simulink model "GalacticSoupFunctional"  (R2025b)
settings: Solver=VariableStepAuto  StartTime=0.0  StopTime=10.0  RelTol=1e-3
settings Model: DataDictionary=GalacticSoupFunctionalInterfaces.sldd  Creator=sarah  LastModifiedBy=sarah

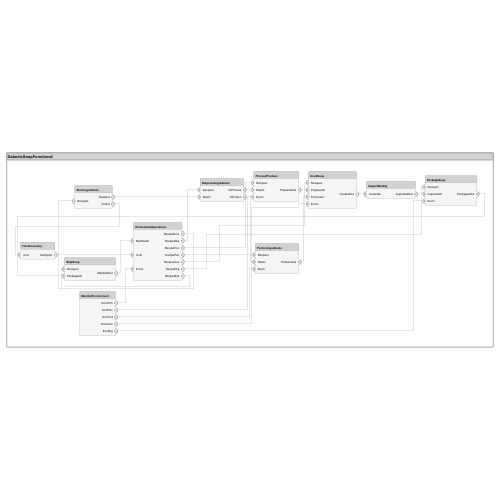
[thumbnail: Simulink's stored preview of the top-level diagram]
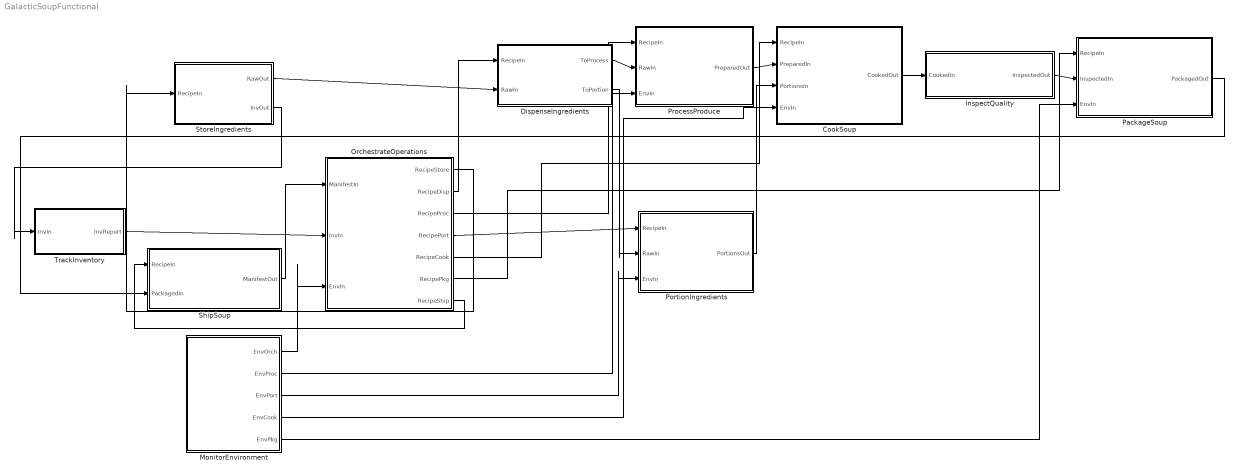
== system GalacticSoupFunctional ==
  CookSoup : Subsystem
      settings: PortSchema="{\"entries\":[{\"content\":{\"headerSize\":26,\"margin\":15,\"minimumSpacing\":25,\"sides\":[{\"content\":{\"connectorIds\":[\"In1\",\"In2\",\"In3\",\"In4\"]},\"type\":\"ConnectorPlacement.EquallySpacedRectSide\",\"uuid\":\"e444b18e-2ceb-4425-8803-e6c31b1fcd82\"},{\"content\":{\"connectorIds\":[\"Out1\"],\"side\":\"RIGHT\"},\"type\":\"ConnectorPlacement.EquallySpacedRectSide\",\"uuid\":\"f4aec6c9-b52d-4884-9c27-2bb07598a416\"},{\"content\":{\"side\":\"TOP\"},\"type\":\"ConnectorPlacement.EquallySpacedRectSide\",\"uuid\":\"1037694d-1bab-41f9-830b-c4a2d0bddcad\"}]},\"type\":\"ConnectorPlacement.EquallySpacedConnector\",\"uuid\":\"fcfa453c-694a-4044-b0a2-73b33e092223\"}],\"packageUris\":[\"http://schema.mathworks.com/mf0/Connector/R2020b\"],\"version\":\"1.0\"}"
  DispenseIngredients : Subsystem
      settings: PortSchema="{\"entries\":[{\"content\":{\"headerSize\":26,\"margin\":15,\"minimumSpacing\":25,\"sides\":[{\"content\":{\"connectorIds\":[\"In1\",\"In2\"]},\"type\":\"ConnectorPlacement.EquallySpacedRectSide\",\"uuid\":\"e444b18e-2ceb-4425-8803-e6c31b1fcd82\"},{\"content\":{\"connectorIds\":[\"Out1\",\"Out2\"],\"side\":\"RIGHT\"},\"type\":\"ConnectorPlacement.EquallySpacedRectSide\",\"uuid\":\"f4aec6c9-b52d-4884-9c27-2bb07598a416\"},{\"content\":{\"side\":\"TOP\"},\"type\":\"ConnectorPlacement.EquallySpacedRectSide\",\"uuid\":\"1037694d-1bab-41f9-830b-c4a2d0bddcad\"}]},\"type\":\"ConnectorPlacement.EquallySpacedConnector\",\"uuid\":\"fcfa453c-694a-4044-b0a2-73b33e092223\"}],\"packageUris\":[\"http://schema.mathworks.com/mf0/Connector/R2020b\"],\"version\":\"1.0\"}"
  InspectQuality : Subsystem
      settings: PortSchema="{\"entries\":[{\"content\":{\"headerSize\":26,\"margin\":15,\"minimumSpacing\":25,\"sides\":[{\"content\":{\"connectorIds\":[\"In1\"]},\"type\":\"ConnectorPlacement.EquallySpacedRectSide\",\"uuid\":\"e444b18e-2ceb-4425-8803-e6c31b1fcd82\"},{\"content\":{\"connectorIds\":[\"Out1\"],\"side\":\"RIGHT\"},\"type\":\"ConnectorPlacement.EquallySpacedRectSide\",\"uuid\":\"f4aec6c9-b52d-4884-9c27-2bb07598a416\"},{\"content\":{\"side\":\"TOP\"},\"type\":\"ConnectorPlacement.EquallySpacedRectSide\",\"uuid\":\"1037694d-1bab-41f9-830b-c4a2d0bddcad\"}]},\"type\":\"ConnectorPlacement.EquallySpacedConnector\",\"uuid\":\"fcfa453c-694a-4044-b0a2-73b33e092223\"}],\"packageUris\":[\"http://schema.mathworks.com/mf0/Connector/R2020b\"],\"version\":\"1.0\"}"
  MonitorEnvironment : Subsystem
      settings: PortSchema="{\"entries\":[{\"content\":{\"headerSize\":26,\"margin\":15,\"minimumSpacing\":25,\"sides\":[{\"content\":{},\"type\":\"ConnectorPlacement.EquallySpacedRectSide\",\"uuid\":\"e444b18e-2ceb-4425-8803-e6c31b1fcd82\"},{\"content\":{\"connectorIds\":[\"Out1\",\"Out2\",\"Out3\",\"Out4\",\"Out5\"],\"side\":\"RIGHT\"},\"type\":\"ConnectorPlacement.EquallySpacedRectSide\",\"uuid\":\"f4aec6c9-b52d-4884-9c27-2bb07598a416\"},{\"content\":{\"side\":\"TOP\"},\"type\":\"ConnectorPlacement.EquallySpacedRectSide\",\"uuid\":\"1037694d-1bab-41f9-830b-c4a2d0bddcad\"}]},\"type\":\"ConnectorPlacement.EquallySpacedConnector\",\"uuid\":\"fcfa453c-694a-4044-b0a2-73b33e092223\"}],\"packageUris\":[\"http://schema.mathworks.com/mf0/Connector/R2020b\"],\"version\":\"1.0\"}"
  OrchestrateOperations : Subsystem
      settings: PortSchema="{\"entries\":[{\"content\":{\"headerSize\":26,\"margin\":15,\"minimumSpacing\":25,\"sides\":[{\"content\":{\"connectorIds\":[\"In1\",\"In2\",\"In3\"]},\"type\":\"ConnectorPlacement.EquallySpacedRectSide\",\"uuid\":\"e444b18e-2ceb-4425-8803-e6c31b1fcd82\"},{\"content\":{\"connectorIds\":[\"Out1\",\"Out2\",\"Out3\",\"Out4\",\"Out5\",\"Out6\",\"Out7\"],\"side\":\"RIGHT\"},\"type\":\"ConnectorPlacement.EquallySpacedRectSide\",\"uuid\":\"f4aec6c9-b52d-4884-9c27-2bb07598a416\"},{\"content\":{\"side\":\"TOP\"},\"type\":\"ConnectorPlacement.EquallySpacedRectSide\",\"uuid\":\"1037694d-1bab-41f9-830b-c4a2d0bddcad\"}]},\"type\":\"ConnectorPlacement.EquallySpacedConnector\",\"uuid\":\"fcfa453c-694a-4044-b0a2-73b33e092223\"}],\"packageUris\":[\"http://schema.mathworks.com/mf0/Connector/R2020b\"],\"version\":\"1.0\"}"
  PackageSoup : Subsystem
      settings: PortSchema="{\"entries\":[{\"content\":{\"headerSize\":26,\"margin\":15,\"minimumSpacing\":25,\"sides\":[{\"content\":{\"connectorIds\":[\"In1\",\"In2\",\"In3\"]},\"type\":\"ConnectorPlacement.EquallySpacedRectSide\",\"uuid\":\"e444b18e-2ceb-4425-8803-e6c31b1fcd82\"},{\"content\":{\"connectorIds\":[\"Out1\"],\"side\":\"RIGHT\"},\"type\":\"ConnectorPlacement.EquallySpacedRectSide\",\"uuid\":\"f4aec6c9-b52d-4884-9c27-2bb07598a416\"},{\"content\":{\"side\":\"TOP\"},\"type\":\"ConnectorPlacement.EquallySpacedRectSide\",\"uuid\":\"1037694d-1bab-41f9-830b-c4a2d0bddcad\"}]},\"type\":\"ConnectorPlacement.EquallySpacedConnector\",\"uuid\":\"fcfa453c-694a-4044-b0a2-73b33e092223\"}],\"packageUris\":[\"http://schema.mathworks.com/mf0/Connector/R2020b\"],\"version\":\"1.0\"}"
  PortionIngredients : Subsystem
      settings: PortSchema="{\"entries\":[{\"content\":{\"headerSize\":26,\"margin\":15,\"minimumSpacing\":25,\"sides\":[{\"content\":{\"connectorIds\":[\"In1\",\"In2\",\"In3\"]},\"type\":\"ConnectorPlacement.EquallySpacedRectSide\",\"uuid\":\"e444b18e-2ceb-4425-8803-e6c31b1fcd82\"},{\"content\":{\"connectorIds\":[\"Out1\"],\"side\":\"RIGHT\"},\"type\":\"ConnectorPlacement.EquallySpacedRectSide\",\"uuid\":\"f4aec6c9-b52d-4884-9c27-2bb07598a416\"},{\"content\":{\"side\":\"TOP\"},\"type\":\"ConnectorPlacement.EquallySpacedRectSide\",\"uuid\":\"1037694d-1bab-41f9-830b-c4a2d0bddcad\"}]},\"type\":\"ConnectorPlacement.EquallySpacedConnector\",\"uuid\":\"fcfa453c-694a-4044-b0a2-73b33e092223\"}],\"packageUris\":[\"http://schema.mathworks.com/mf0/Connector/R2020b\"],\"version\":\"1.0\"}"
  ProcessProduce : Subsystem
      settings: PortSchema="{\"entries\":[{\"content\":{\"headerSize\":26,\"margin\":15,\"minimumSpacing\":25,\"sides\":[{\"content\":{\"connectorIds\":[\"In1\",\"In2\",\"In3\"]},\"type\":\"ConnectorPlacement.EquallySpacedRectSide\",\"uuid\":\"e444b18e-2ceb-4425-8803-e6c31b1fcd82\"},{\"content\":{\"connectorIds\":[\"Out1\"],\"side\":\"RIGHT\"},\"type\":\"ConnectorPlacement.EquallySpacedRectSide\",\"uuid\":\"f4aec6c9-b52d-4884-9c27-2bb07598a416\"},{\"content\":{\"side\":\"TOP\"},\"type\":\"ConnectorPlacement.EquallySpacedRectSide\",\"uuid\":\"1037694d-1bab-41f9-830b-c4a2d0bddcad\"}]},\"type\":\"ConnectorPlacement.EquallySpacedConnector\",\"uuid\":\"fcfa453c-694a-4044-b0a2-73b33e092223\"}],\"packageUris\":[\"http://schema.mathworks.com/mf0/Connector/R2020b\"],\"version\":\"1.0\"}"
  ShipSoup : Subsystem
      settings: PortSchema="{\"entries\":[{\"content\":{\"headerSize\":26,\"margin\":15,\"minimumSpacing\":25,\"sides\":[{\"content\":{\"connectorIds\":[\"In1\",\"In2\"]},\"type\":\"ConnectorPlacement.EquallySpacedRectSide\",\"uuid\":\"e444b18e-2ceb-4425-8803-e6c31b1fcd82\"},{\"content\":{\"connectorIds\":[\"Out1\"],\"side\":\"RIGHT\"},\"type\":\"ConnectorPlacement.EquallySpacedRectSide\",\"uuid\":\"f4aec6c9-b52d-4884-9c27-2bb07598a416\"},{\"content\":{\"side\":\"TOP\"},\"type\":\"ConnectorPlacement.EquallySpacedRectSide\",\"uuid\":\"1037694d-1bab-41f9-830b-c4a2d0bddcad\"}]},\"type\":\"ConnectorPlacement.EquallySpacedConnector\",\"uuid\":\"fcfa453c-694a-4044-b0a2-73b33e092223\"}],\"packageUris\":[\"http://schema.mathworks.com/mf0/Connector/R2020b\"],\"version\":\"1.0\"}"
  StoreIngredients : Subsystem
      settings: PortSchema="{\"entries\":[{\"content\":{\"headerSize\":26,\"margin\":15,\"minimumSpacing\":25,\"sides\":[{\"content\":{\"connectorIds\":[\"In1\"]},\"type\":\"ConnectorPlacement.EquallySpacedRectSide\",\"uuid\":\"e444b18e-2ceb-4425-8803-e6c31b1fcd82\"},{\"content\":{\"connectorIds\":[\"Out1\",\"Out2\"],\"side\":\"RIGHT\"},\"type\":\"ConnectorPlacement.EquallySpacedRectSide\",\"uuid\":\"f4aec6c9-b52d-4884-9c27-2bb07598a416\"},{\"content\":{\"side\":\"TOP\"},\"type\":\"ConnectorPlacement.EquallySpacedRectSide\",\"uuid\":\"1037694d-1bab-41f9-830b-c4a2d0bddcad\"}]},\"type\":\"ConnectorPlacement.EquallySpacedConnector\",\"uuid\":\"fcfa453c-694a-4044-b0a2-73b33e092223\"}],\"packageUris\":[\"http://schema.mathworks.com/mf0/Connector/R2020b\"],\"version\":\"1.0\"}"
  TrackInventory : Subsystem
      settings: PortSchema="{\"entries\":[{\"content\":{\"headerSize\":26,\"margin\":15,\"minimumSpacing\":25,\"sides\":[{\"content\":{\"connectorIds\":[\"In1\"]},\"type\":\"ConnectorPlacement.EquallySpacedRectSide\",\"uuid\":\"e444b18e-2ceb-4425-8803-e6c31b1fcd82\"},{\"content\":{\"connectorIds\":[\"Out1\"],\"side\":\"RIGHT\"},\"type\":\"ConnectorPlacement.EquallySpacedRectSide\",\"uuid\":\"f4aec6c9-b52d-4884-9c27-2bb07598a416\"},{\"content\":{\"side\":\"TOP\"},\"type\":\"ConnectorPlacement.EquallySpacedRectSide\",\"uuid\":\"1037694d-1bab-41f9-830b-c4a2d0bddcad\"}]},\"type\":\"ConnectorPlacement.EquallySpacedConnector\",\"uuid\":\"fcfa453c-694a-4044-b0a2-73b33e092223\"}],\"packageUris\":[\"http://schema.mathworks.com/mf0/Connector/R2020b\"],\"version\":\"1.0\"}"
  wires:
  MonitorEnvironment/4(EnvCook) -> CookSoup/4(EnvIn)
  MonitorEnvironment/3(EnvPort) -> PortionIngredients/3(EnvIn)
  MonitorEnvironment/2(EnvProc) -> ProcessProduce/3(EnvIn)
  MonitorEnvironment/1(EnvOrch) -> OrchestrateOperations/3(EnvIn)
  TrackInventory/1(InvReport) -> OrchestrateOperations/2(InvIn)
  StoreIngredients/1(RawOut) -> DispenseIngredients/2(RawIn)
  ShipSoup/1(ManifestOut) -> OrchestrateOperations/1(ManifestIn)
  StoreIngredients/2(InvOut) -> TrackInventory/1(InvIn)
  MonitorEnvironment/5(EnvPkg) -> PackageSoup/3(EnvIn)
  OrchestrateOperations/1(RecipeStore) -> StoreIngredients/1(RecipeIn)
  OrchestrateOperations/2(RecipeDisp) -> DispenseIngredients/1(RecipeIn)
  OrchestrateOperations/3(RecipeProc) -> ProcessProduce/1(RecipeIn)
  OrchestrateOperations/4(RecipePort) -> PortionIngredients/1(RecipeIn)
  OrchestrateOperations/5(RecipeCook) -> CookSoup/1(RecipeIn)
  OrchestrateOperations/6(RecipePkg) -> PackageSoup/1(RecipeIn)
  OrchestrateOperations/7(RecipeShip) -> ShipSoup/1(RecipeIn)
  DispenseIngredients/1(ToProcess) -> ProcessProduce/2(RawIn)
  DispenseIngredients/2(ToPortion) -> PortionIngredients/2(RawIn)
  ProcessProduce/1(PreparedOut) -> CookSoup/2(PreparedIn)
  PortionIngredients/1(PortionsOut) -> CookSoup/3(PortionsIn)
  CookSoup/1(CookedOut) -> InspectQuality/1(CookedIn)
  InspectQuality/1(InspectedOut) -> PackageSoup/2(InspectedIn)
  PackageSoup/1(PackagedOut) -> ShipSoup/2(PackagedIn)

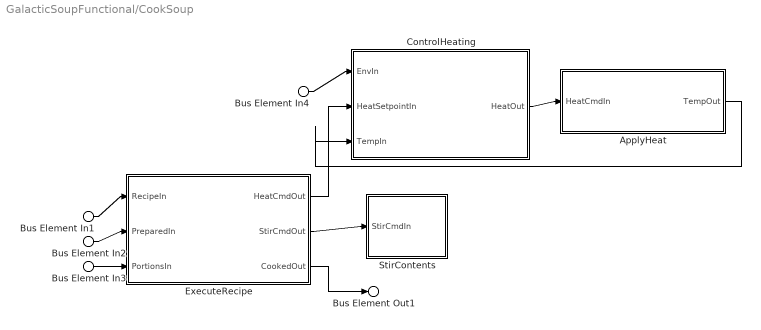
== system GalacticSoupFunctional/CookSoup ==
  Bus Element In1 : Inport  PortName=RecipeIn
  Bus Element In2 : Inport  Port=2  PortName=PreparedIn
  Bus Element In3 : Inport  Port=3  PortName=PortionsIn
  Bus Element In4 : Inport  Port=4  PortName=EnvIn
  ApplyHeat : Subsystem
      settings: PortSchema="{\"entries\":[{\"content\":{\"headerSize\":26,\"margin\":15,\"minimumSpacing\":25,\"sides\":[{\"content\":{\"connectorIds\":[\"In1\"]},\"type\":\"ConnectorPlacement.EquallySpacedRectSide\",\"uuid\":\"e444b18e-2ceb-4425-8803-e6c31b1fcd82\"},{\"content\":{\"connectorIds\":[\"Out1\"],\"side\":\"RIGHT\"},\"type\":\"ConnectorPlacement.EquallySpacedRectSide\",\"uuid\":\"f4aec6c9-b52d-4884-9c27-2bb07598a416\"},{\"content\":{\"side\":\"TOP\"},\"type\":\"ConnectorPlacement.EquallySpacedRectSide\",\"uuid\":\"1037694d-1bab-41f9-830b-c4a2d0bddcad\"}]},\"type\":\"ConnectorPlacement.EquallySpacedConnector\",\"uuid\":\"fcfa453c-694a-4044-b0a2-73b33e092223\"}],\"packageUris\":[\"http://schema.mathworks.com/mf0/Connector/R2020b\"],\"version\":\"1.0\"}"
  ControlHeating : Subsystem
      settings: PortSchema="{\"entries\":[{\"content\":{\"headerSize\":26,\"margin\":15,\"minimumSpacing\":25,\"sides\":[{\"content\":{\"connectorIds\":[\"In1\",\"In2\",\"In3\"]},\"type\":\"ConnectorPlacement.EquallySpacedRectSide\",\"uuid\":\"e444b18e-2ceb-4425-8803-e6c31b1fcd82\"},{\"content\":{\"connectorIds\":[\"Out1\"],\"side\":\"RIGHT\"},\"type\":\"ConnectorPlacement.EquallySpacedRectSide\",\"uuid\":\"f4aec6c9-b52d-4884-9c27-2bb07598a416\"},{\"content\":{\"side\":\"TOP\"},\"type\":\"ConnectorPlacement.EquallySpacedRectSide\",\"uuid\":\"1037694d-1bab-41f9-830b-c4a2d0bddcad\"}]},\"type\":\"ConnectorPlacement.EquallySpacedConnector\",\"uuid\":\"fcfa453c-694a-4044-b0a2-73b33e092223\"}],\"packageUris\":[\"http://schema.mathworks.com/mf0/Connector/R2020b\"],\"version\":\"1.0\"}"
  ExecuteRecipe : Subsystem
      settings: PortSchema="{\"entries\":[{\"content\":{\"headerSize\":26,\"margin\":15,\"minimumSpacing\":25,\"sides\":[{\"content\":{\"connectorIds\":[\"In1\",\"In2\",\"In3\"]},\"type\":\"ConnectorPlacement.EquallySpacedRectSide\",\"uuid\":\"e444b18e-2ceb-4425-8803-e6c31b1fcd82\"},{\"content\":{\"connectorIds\":[\"Out1\",\"Out2\",\"Out3\"],\"side\":\"RIGHT\"},\"type\":\"ConnectorPlacement.EquallySpacedRectSide\",\"uuid\":\"f4aec6c9-b52d-4884-9c27-2bb07598a416\"},{\"content\":{\"side\":\"TOP\"},\"type\":\"ConnectorPlacement.EquallySpacedRectSide\",\"uuid\":\"1037694d-1bab-41f9-830b-c4a2d0bddcad\"}]},\"type\":\"ConnectorPlacement.EquallySpacedConnector\",\"uuid\":\"fcfa453c-694a-4044-b0a2-73b33e092223\"}],\"packageUris\":[\"http://schema.mathworks.com/mf0/Connector/R2020b\"],\"version\":\"1.0\"}"
  StirContents : Subsystem
      settings: PortSchema="{\"entries\":[{\"content\":{\"headerSize\":26,\"margin\":15,\"minimumSpacing\":25,\"sides\":[{\"content\":{\"connectorIds\":[\"In1\"]},\"type\":\"ConnectorPlacement.EquallySpacedRectSide\",\"uuid\":\"e444b18e-2ceb-4425-8803-e6c31b1fcd82\"},{\"content\":{\"side\":\"RIGHT\"},\"type\":\"ConnectorPlacement.EquallySpacedRectSide\",\"uuid\":\"f4aec6c9-b52d-4884-9c27-2bb07598a416\"},{\"content\":{\"side\":\"TOP\"},\"type\":\"ConnectorPlacement.EquallySpacedRectSide\",\"uuid\":\"1037694d-1bab-41f9-830b-c4a2d0bddcad\"}]},\"type\":\"ConnectorPlacement.EquallySpacedConnector\",\"uuid\":\"fcfa453c-694a-4044-b0a2-73b33e092223\"}],\"packageUris\":[\"http://schema.mathworks.com/mf0/Connector/R2020b\"],\"version\":\"1.0\"}"
  Bus Element Out1 : Outport  PortName=CookedOut
  wires:
  Bus Element In1/1 -> ExecuteRecipe/1(RecipeIn)
  Bus Element In3/1 -> ExecuteRecipe/3(PortionsIn)
  Bus Element In2/1 -> ExecuteRecipe/2(PreparedIn)
  Bus Element In4/1 -> ControlHeating/1(EnvIn)
  ExecuteRecipe/1(HeatCmdOut) -> ControlHeating/2(HeatSetpointIn)
  ControlHeating/1(HeatOut) -> ApplyHeat/1(HeatCmdIn)
  ExecuteRecipe/3(CookedOut) -> Bus Element Out1/1
  ExecuteRecipe/2(StirCmdOut) -> StirContents/1(StirCmdIn)
  ApplyHeat/1(TempOut) -> ControlHeating/3(TempIn)

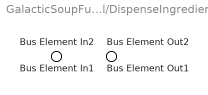
== system GalacticSoupFunctional/DispenseIngredients ==
  Bus Element In1 : Inport  PortName=RecipeIn
  Bus Element In2 : Inport  Port=2  PortName=RawIn
  Bus Element Out1 : Outport  PortName=ToProcess
  Bus Element Out2 : Outport  Port=2  PortName=ToPortion

== system GalacticSoupFunctional/InspectQuality ==
  Bus Element In1 : Inport  PortName=CookedIn
  Bus Element Out1 : Outport  PortName=InspectedOut

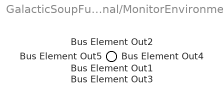
== system GalacticSoupFunctional/MonitorEnvironment ==
  Bus Element Out1 : Outport  PortName=EnvOrch
  Bus Element Out2 : Outport  Port=2  PortName=EnvProc
  Bus Element Out3 : Outport  Port=3  PortName=EnvPort
  Bus Element Out4 : Outport  Port=4  PortName=EnvCook
  Bus Element Out5 : Outport  Port=5  PortName=EnvPkg

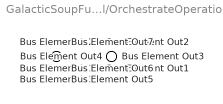
== system GalacticSoupFunctional/OrchestrateOperations ==
  Bus Element In1 : Inport  PortName=ManifestIn
  Bus Element In2 : Inport  Port=2  PortName=InvIn
  Bus Element In3 : Inport  Port=3  PortName=EnvIn
  Bus Element Out1 : Outport  PortName=RecipeStore
  Bus Element Out2 : Outport  Port=2  PortName=RecipeDisp
  Bus Element Out3 : Outport  Port=3  PortName=RecipeProc
  Bus Element Out4 : Outport  Port=4  PortName=RecipePort
  Bus Element Out5 : Outport  Port=5  PortName=RecipeCook
  Bus Element Out6 : Outport  Port=6  PortName=RecipePkg
  Bus Element Out7 : Outport  Port=7  PortName=RecipeShip

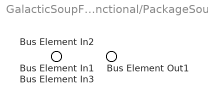
== system GalacticSoupFunctional/PackageSoup ==
  Bus Element In1 : Inport  PortName=RecipeIn
  Bus Element In2 : Inport  Port=2  PortName=InspectedIn
  Bus Element In3 : Inport  Port=3  PortName=EnvIn
  Bus Element Out1 : Outport  PortName=PackagedOut

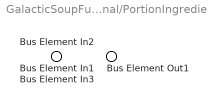
== system GalacticSoupFunctional/PortionIngredients ==
  Bus Element In1 : Inport  PortName=RecipeIn
  Bus Element In2 : Inport  Port=2  PortName=RawIn
  Bus Element In3 : Inport  Port=3  PortName=EnvIn
  Bus Element Out1 : Outport  PortName=PortionsOut

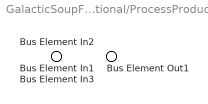
== system GalacticSoupFunctional/ProcessProduce ==
  Bus Element In1 : Inport  PortName=RecipeIn
  Bus Element In2 : Inport  Port=2  PortName=RawIn
  Bus Element In3 : Inport  Port=3  PortName=EnvIn
  Bus Element Out1 : Outport  PortName=PreparedOut

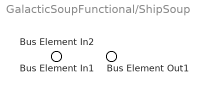
== system GalacticSoupFunctional/ShipSoup ==
  Bus Element In1 : Inport  PortName=RecipeIn
  Bus Element In2 : Inport  Port=2  PortName=PackagedIn
  Bus Element Out1 : Outport  PortName=ManifestOut

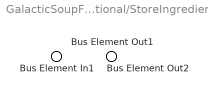
== system GalacticSoupFunctional/StoreIngredients ==
  Bus Element In1 : Inport  PortName=RecipeIn
  Bus Element Out1 : Outport  PortName=RawOut
  Bus Element Out2 : Outport  Port=2  PortName=InvOut

== system GalacticSoupFunctional/TrackInventory ==
  Bus Element In1 : Inport  PortName=InvIn
  Bus Element Out1 : Outport  PortName=InvReport

== system GalacticSoupFunctional/CookSoup/ApplyHeat ==
  Bus Element In1 : Inport  PortName=HeatCmdIn
  Bus Element Out1 : Outport  PortName=TempOut

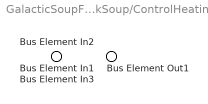
== system GalacticSoupFunctional/CookSoup/ControlHeating ==
  Bus Element In1 : Inport  PortName=EnvIn
  Bus Element In2 : Inport  Port=2  PortName=HeatSetpointIn
  Bus Element In3 : Inport  Port=3  PortName=TempIn
  Bus Element Out1 : Outport  PortName=HeatOut

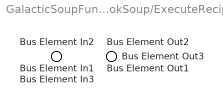
== system GalacticSoupFunctional/CookSoup/ExecuteRecipe ==
  Bus Element In1 : Inport  PortName=RecipeIn
  Bus Element In2 : Inport  Port=2  PortName=PreparedIn
  Bus Element In3 : Inport  Port=3  PortName=PortionsIn
  Bus Element Out1 : Outport  PortName=HeatCmdOut
  Bus Element Out2 : Outport  Port=2  PortName=StirCmdOut
  Bus Element Out3 : Outport  Port=3  PortName=CookedOut

== system GalacticSoupFunctional/CookSoup/StirContents ==
  Bus Element In1 : Inport  PortName=StirCmdIn
